simulink library "AFS_MasterFeature"  (R2020b)
settings: Solver=FixedStepDiscrete  StartTime=0.0  StopTime=10.0  FixedStep=SampleTime  RelTol=1e-3
undefined symbols (not defined in the file): C_AFS_Thr_Speed_HB_HS_OFF, C_AFS_Thr_Speed_HB_HS_ON, C_F_SpeedCountry2Town, C_F_SpeedPed2Town, C_F_SpeedTown2Country, C_F_SpeedTown2Ped, C_F_Time2WaitAFS, C_ParkingSpeedThrAct, C_SpeedCountry2MW, C_SpeedMW2Country, C_TeAfsMaster, C_TempoPark, N_E_AdverseWeather, N_E_Country, N_E_Foggy, N_E_HBHighSpeed, N_E_HBLowSpeed, N_E_Motorway, N_E_NoFunction, N_E_Pedestrian, N_E_TouristMode, N_E_Town, N_LIGHT_NIGHT, N_ManeuverMode
settings Model: Creator=hhamlaou  LastModifiedBy=smettupa
settings DataIOCC: ReturnWorkspaceOutputs=off
settings DebuggingCC: ArithmeticOperatorsInVariantConditions=warning
settings SFSimCC: SimUseLocalCustomCode=off  CustomCodeUndefinedFunction=UseInterfaceOnly
settings RTWCC: RTWUseLocalCustomCode=off

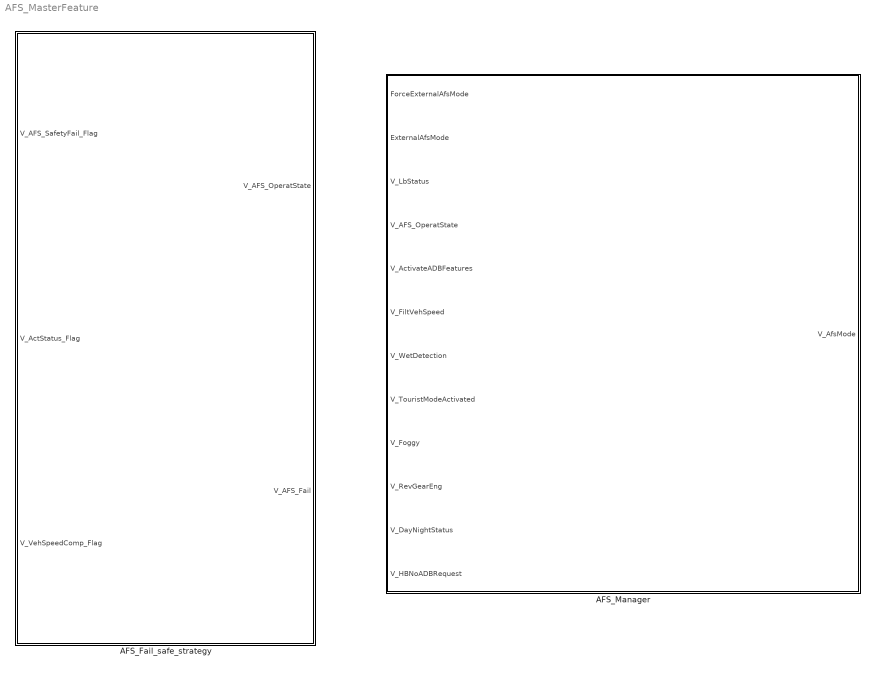
== system AFS_MasterFeature ==
  AFS_Fail_safe_strategy : Stateflow chart  TreatAsAtomicUnit=on
  AFS_Manager : Subsystem  Description=AFS_Subsystem

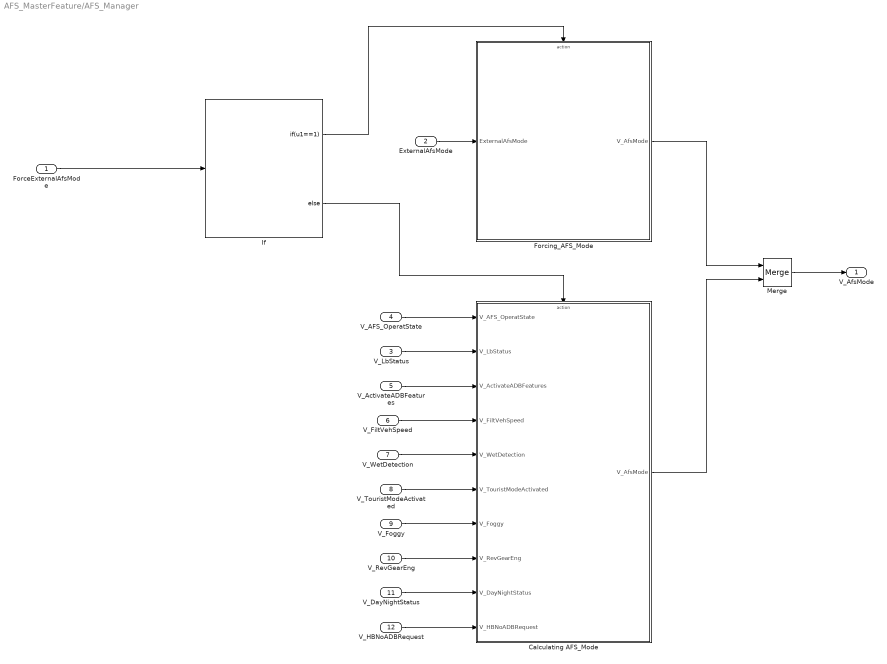
== system AFS_MasterFeature/AFS_Manager ==
  ForceExternalAfsMode : Inport
  ExternalAfsMode : Inport  Port=2
  V_LbStatus : Inport  Port=3
  V_AFS_OperatState : Inport  Port=4
  V_ActivateADBFeatures : Inport  Port=5
  V_FiltVehSpeed : Inport  Port=6
  V_WetDetection : Inport  Port=7
  V_TouristModeActivated : Inport  Port=8
  V_Foggy : Inport  Port=9
  V_RevGearEng : Inport  Port=10
  V_DayNightStatus : Inport  Port=11
  V_HBNoADBRequest : Inport  Port=12
  "Calculating AFS_Mode " : Subsystem  TreatAsAtomicUnit=on
  Forcing_AFS_Mode : Subsystem  TreatAsAtomicUnit=on
  If : If  IfExpression=u1==1
  Merge : Merge
  V_AfsMode : Outport
  wires:
  ForceExternalAfsMode/1 -> If/1
  Forcing_AFS_Mode/1(V_AfsMode) -> Merge/1
  "Calculating AFS_Mode "/1(V_AfsMode) -> Merge/2
  Merge/1 -> V_AfsMode/1
  ExternalAfsMode/1 -> Forcing_AFS_Mode/1(ExternalAfsMode)
  V_LbStatus/1 -> "Calculating AFS_Mode "/2(V_LbStatus)
  V_AFS_OperatState/1 -> "Calculating AFS_Mode "/1(V_AFS_OperatState)
  V_ActivateADBFeatures/1 -> "Calculating AFS_Mode "/3(V_ActivateADBFeatures)
  V_FiltVehSpeed/1 -> "Calculating AFS_Mode "/4(V_FiltVehSpeed)
  V_WetDetection/1 -> "Calculating AFS_Mode "/5(V_WetDetection)
  V_TouristModeActivated/1 -> "Calculating AFS_Mode "/6(V_TouristModeActivated)
  V_Foggy/1 -> "Calculating AFS_Mode "/7(V_Foggy)
  V_RevGearEng/1 -> "Calculating AFS_Mode "/8(V_RevGearEng)
  V_DayNightStatus/1 -> "Calculating AFS_Mode "/9(V_DayNightStatus)
  If/1 -> Forcing_AFS_Mode/Action
  V_HBNoADBRequest/1 -> "Calculating AFS_Mode "/10(V_HBNoADBRequest)
  If/2 -> "Calculating AFS_Mode "/Action

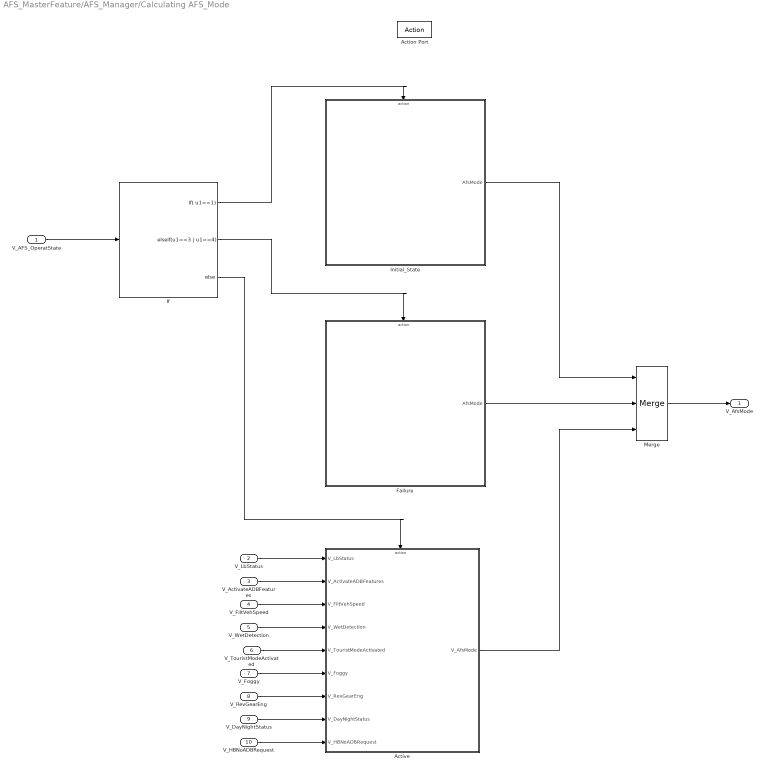
== system AFS_MasterFeature/AFS_Manager/Calculating AFS_Mode  ==
  V_AFS_OperatState : Inport
  V_LbStatus : Inport  Port=2
  V_ActivateADBFeatures : Inport  Port=3
  V_FiltVehSpeed : Inport  Port=4
  V_WetDetection : Inport  Port=5
  V_TouristModeActivated : Inport  Port=6
  V_Foggy : Inport  Port=7
  V_RevGearEng : Inport  Port=8
  V_DayNightStatus : Inport  Port=9
  V_HBNoADBRequest : Inport  Port=10
  Action Port : ActionPort
  Active : Subsystem  TreatAsAtomicUnit=on
  Failure : Subsystem  TreatAsAtomicUnit=on
  If : If  IfExpression=u1==1  ElseIfExpressions=u1==3 | u1==4
  Initial_State : Subsystem  TreatAsAtomicUnit=on
  Merge : Merge  Inputs=3
  V_AfsMode : Outport
  wires:
  V_AFS_OperatState/1 -> If/1
  If/2 -> Failure/Action
  If/3 -> Active/Action
  Failure/1(AfsMode) -> Merge/2
  Initial_State/1(AfsMode) -> Merge/1
  Active/1(V_AfsMode) -> Merge/3
  Merge/1 -> V_AfsMode/1
  V_ActivateADBFeatures/1 -> Active/2(V_ActivateADBFeatures)
  V_LbStatus/1 -> Active/1(V_LbStatus)
  V_FiltVehSpeed/1 -> Active/3(V_FiltVehSpeed)
  V_WetDetection/1 -> Active/4(V_WetDetection)
  V_TouristModeActivated/1 -> Active/5(V_TouristModeActivated)
  V_Foggy/1 -> Active/6(V_Foggy)
  V_RevGearEng/1 -> Active/7(V_RevGearEng)
  V_DayNightStatus/1 -> Active/8(V_DayNightStatus)
  V_HBNoADBRequest/1 -> Active/9(V_HBNoADBRequest)
  If/1 -> Initial_State/Action

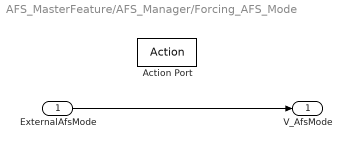
== system AFS_MasterFeature/AFS_Manager/Forcing_AFS_Mode ==
  ExternalAfsMode : Inport
  Action Port : ActionPort
  V_AfsMode : Outport
  wires:
  ExternalAfsMode/1 -> V_AfsMode/1

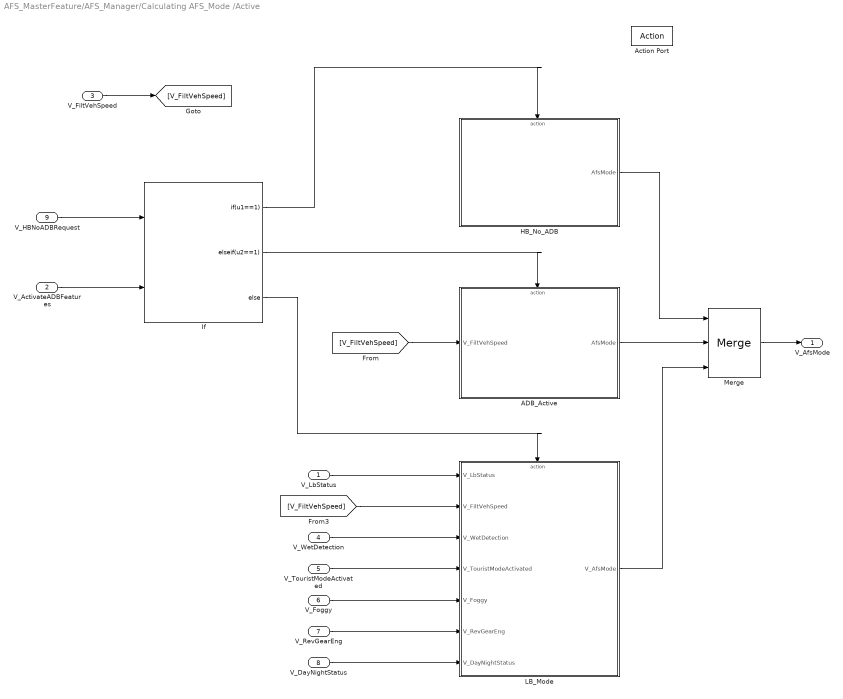
== system AFS_MasterFeature/AFS_Manager/Calculating AFS_Mode /Active ==
  V_LbStatus : Inport
  V_ActivateADBFeatures : Inport  Port=2
  V_FiltVehSpeed : Inport  Port=3
  V_WetDetection : Inport  Port=4
  V_TouristModeActivated : Inport  Port=5
  V_Foggy : Inport  Port=6
  V_RevGearEng : Inport  Port=7
  V_DayNightStatus : Inport  Port=8
  V_HBNoADBRequest : Inport  Port=9
  Action Port : ActionPort
  ADB_Active : Subsystem  TreatAsAtomicUnit=on
  HB_No_ADB : Subsystem  TreatAsAtomicUnit=on
  If : If  NumInputs=2  IfExpression=u1==1  ElseIfExpressions=u2==1
  LB_Mode : Subsystem  TreatAsAtomicUnit=on
  Merge : Merge  Inputs=3
  V_AfsMode : Outport
  wires:
  V_FiltVehSpeed/1 -> [V_FiltVehSpeed]
  V_HBNoADBRequest/1 -> If/1
  If/1 -> HB_No_ADB/Action
  V_ActivateADBFeatures/1 -> If/2
  If/2 -> ADB_Active/Action
  If/3 -> LB_Mode/Action
  ADB_Active/1(AfsMode) -> Merge/2
  HB_No_ADB/1(AfsMode) -> Merge/1
  LB_Mode/1(V_AfsMode) -> Merge/3
  [V_FiltVehSpeed] -> ADB_Active/1(V_FiltVehSpeed)
  Merge/1 -> V_AfsMode/1
  V_LbStatus/1 -> LB_Mode/1(V_LbStatus)
  [V_FiltVehSpeed] -> LB_Mode/2(V_FiltVehSpeed)
  V_WetDetection/1 -> LB_Mode/3(V_WetDetection)
  V_TouristModeActivated/1 -> LB_Mode/4(V_TouristModeActivated)
  V_Foggy/1 -> LB_Mode/5(V_Foggy)
  V_RevGearEng/1 -> LB_Mode/6(V_RevGearEng)
  V_DayNightStatus/1 -> LB_Mode/7(V_DayNightStatus)

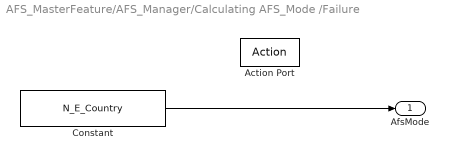
== system AFS_MasterFeature/AFS_Manager/Calculating AFS_Mode /Failure ==
  Action Port : ActionPort
  Constant : Constant  Value=N_E_Country
  AfsMode : Outport
  wires:
  Constant/1 -> AfsMode/1

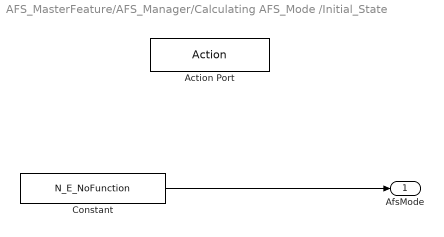
== system AFS_MasterFeature/AFS_Manager/Calculating AFS_Mode /Initial_State ==
  Action Port : ActionPort
  Constant : Constant  Value=N_E_NoFunction
  AfsMode : Outport
  wires:
  Constant/1 -> AfsMode/1

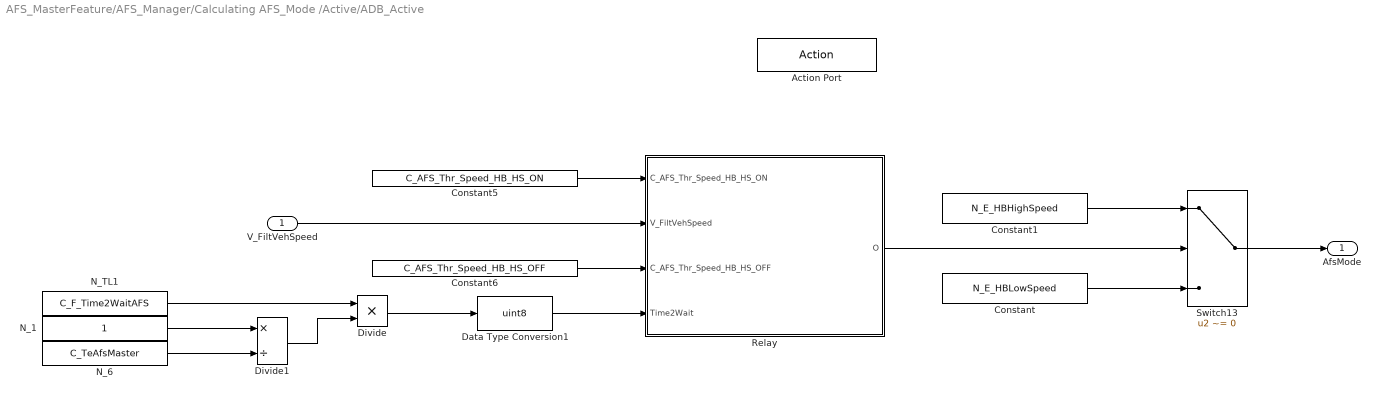
== system AFS_MasterFeature/AFS_Manager/Calculating AFS_Mode /Active/ADB_Active ==
  V_FiltVehSpeed : Inport
  Action Port : ActionPort
  Constant : Constant  Value=N_E_HBLowSpeed
  Constant1 : Constant  Value=N_E_HBHighSpeed
  Constant5 : Constant  Value=C_AFS_Thr_Speed_HB_HS_ON
  Constant6 : Constant  Value=C_AFS_Thr_Speed_HB_HS_OFF
  Data Type Conversion1 : DataTypeConversion  OutDataTypeStr=uint8
  Divide : Product  Inputs=**
  Divide1 : Product  Inputs=*/  OutDataTypeStr=uint8
  N_1 : Constant  OutDataTypeStr=uint8
  N_6 : Constant  Value=C_TeAfsMaster
  N_TL1 : Constant  Value=C_F_Time2WaitAFS
  Relay : Stateflow chart  TreatAsAtomicUnit=on
  Switch13 : Switch  Criteria=u2 ~= 0
  AfsMode : Outport
  wires:
  V_FiltVehSpeed/1 -> Relay/2(V_FiltVehSpeed)
  Data Type Conversion1/1 -> Relay/4(Time2Wait)
  Constant5/1 -> Relay/1(C_AFS_Thr_Speed_HB_HS_ON)
  Constant6/1 -> Relay/3(C_AFS_Thr_Speed_HB_HS_OFF)
  Relay/1(O) -> Switch13/2
  Constant1/1 -> Switch13/1
  Constant/1 -> Switch13/3
  Switch13/1 -> AfsMode/1
  N_1/1 -> Divide1/1
  Divide/1 -> Data Type Conversion1/1
  N_TL1/1 -> Divide/1
  Divide1/1 -> Divide/2
  N_6/1 -> Divide1/2

== system AFS_MasterFeature/AFS_Manager/Calculating AFS_Mode /Active/HB_No_ADB ==
  Action Port : ActionPort
  Constant : Constant  Value=N_E_HBLowSpeed
  AfsMode : Outport
  wires:
  Constant/1 -> AfsMode/1

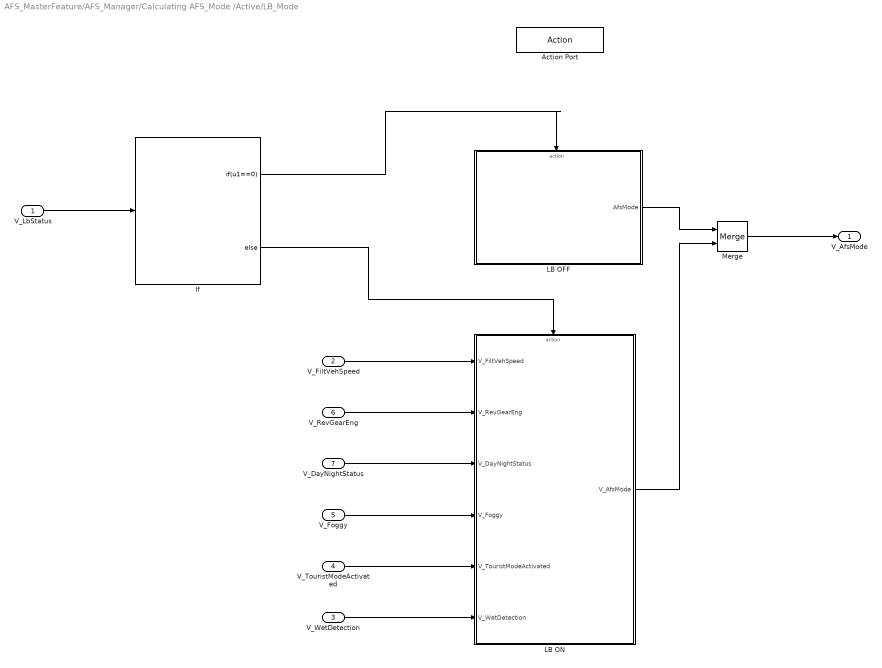
== system AFS_MasterFeature/AFS_Manager/Calculating AFS_Mode /Active/LB_Mode ==
  V_LbStatus : Inport
  V_FiltVehSpeed : Inport  Port=2
  V_WetDetection : Inport  Port=3
  V_TouristModeActivated : Inport  Port=4
  V_Foggy : Inport  Port=5
  V_RevGearEng : Inport  Port=6
  V_DayNightStatus : Inport  Port=7
  Action Port : ActionPort
  If : If  IfExpression=u1==0
  LB OFF : Subsystem  TreatAsAtomicUnit=on
  LB ON : Subsystem  TreatAsAtomicUnit=on
  Merge : Merge
  V_AfsMode : Outport
  wires:
  If/1 -> LB OFF/Action
  If/2 -> LB ON/Action
  LB OFF/1(AfsMode) -> Merge/1
  LB ON/1(V_AfsMode) -> Merge/2
  Merge/1 -> V_AfsMode/1
  V_FiltVehSpeed/1 -> LB ON/1(V_FiltVehSpeed)
  V_LbStatus/1 -> If/1
  V_RevGearEng/1 -> LB ON/2(V_RevGearEng)
  V_DayNightStatus/1 -> LB ON/3(V_DayNightStatus)
  V_Foggy/1 -> LB ON/4(V_Foggy)
  V_TouristModeActivated/1 -> LB ON/5(V_TouristModeActivated)
  V_WetDetection/1 -> LB ON/6(V_WetDetection)

== system AFS_MasterFeature/AFS_Manager/Calculating AFS_Mode /Active/LB_Mode/LB OFF ==
  Action Port : ActionPort
  Constant : Constant  Value=N_E_NoFunction
  AfsMode : Outport
  wires:
  Constant/1 -> AfsMode/1

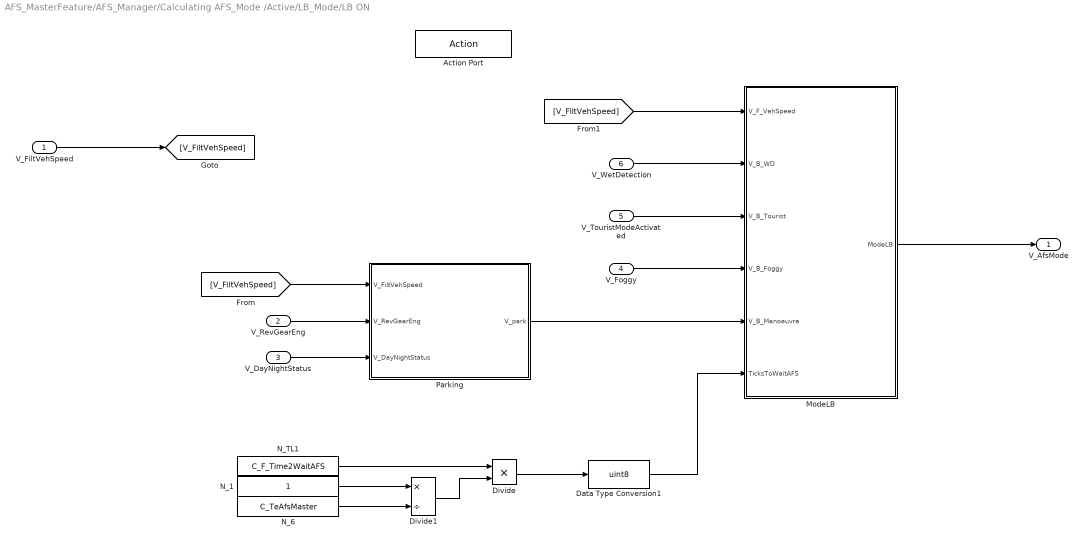
== system AFS_MasterFeature/AFS_Manager/Calculating AFS_Mode /Active/LB_Mode/LB ON ==
  V_FiltVehSpeed : Inport
  V_RevGearEng : Inport  Port=2
  V_DayNightStatus : Inport  Port=3
  V_Foggy : Inport  Port=4
  V_TouristModeActivated : Inport  Port=5
  V_WetDetection : Inport  Port=6
  Action Port : ActionPort
  Data Type Conversion1 : DataTypeConversion  OutDataTypeStr=uint8
  Divide : Product  Inputs=**
  Divide1 : Product  Inputs=*/  OutDataTypeStr=uint8
  ModeLB : Subsystem  Description=ModeLB
  N_1 : Constant  OutDataTypeStr=uint8
  N_6 : Constant  Value=C_TeAfsMaster
  N_TL1 : Constant  Value=C_F_Time2WaitAFS
  Parking : Subsystem  TreatAsAtomicUnit=on
  V_AfsMode : Outport
  wires:
  Parking/1(V_park) -> ModeLB/5(V_B_Manoeuvre)
  N_TL1/1 -> Divide/1
  Data Type Conversion1/1 -> ModeLB/6(TicksToWaitAFS)
  N_6/1 -> Divide1/2
  Divide/1 -> Data Type Conversion1/1
  Divide1/1 -> Divide/2
  N_1/1 -> Divide1/1
  ModeLB/1(ModeLB) -> V_AfsMode/1
  V_RevGearEng/1 -> Parking/2(V_RevGearEng)
  V_DayNightStatus/1 -> Parking/3(V_DayNightStatus)
  V_Foggy/1 -> ModeLB/4(V_B_Foggy)
  V_TouristModeActivated/1 -> ModeLB/3(V_B_Tourist)
  V_WetDetection/1 -> ModeLB/2(V_B_WD)
  V_FiltVehSpeed/1 -> [V_FiltVehSpeed]
  [V_FiltVehSpeed] -> Parking/1(V_FiltVehSpeed)
  [V_FiltVehSpeed] -> ModeLB/1(V_F_VehSpeed)

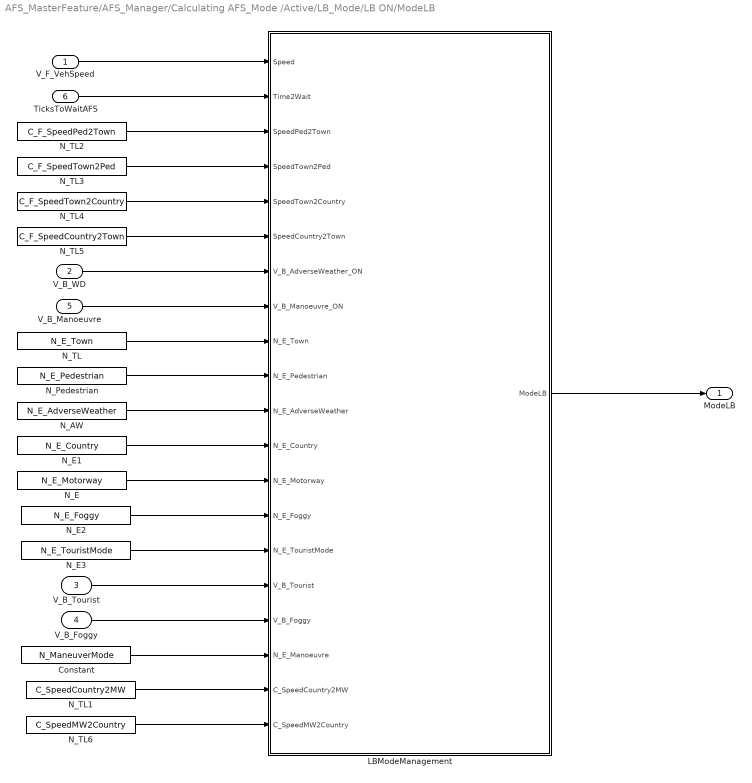
== system AFS_MasterFeature/AFS_Manager/Calculating AFS_Mode /Active/LB_Mode/LB ON/ModeLB ==
  V_F_VehSpeed : Inport
  V_B_WD : Inport  Port=2
  V_B_Tourist : Inport  Port=3
  V_B_Foggy : Inport  Port=4
  V_B_Manoeuvre : Inport  Port=5
  TicksToWaitAFS : Inport  Port=6
      settings: AttributesFormatString=%<OutDataTypeStr>
  Constant : Constant  Value=N_ManeuverMode
  LBModeManagement : Stateflow chart
  N_AW : Constant  Value=N_E_AdverseWeather
  N_E : Constant  Value=N_E_Motorway
  N_E1 : Constant  Value=N_E_Country
  N_E2 : Constant  Value=N_E_Foggy
  N_E3 : Constant  Value=N_E_TouristMode
  N_Pedestrian : Constant  Value=N_E_Pedestrian
  N_TL : Constant  Value=N_E_Town
  N_TL1 : Constant  Value=C_SpeedCountry2MW
  N_TL2 : Constant  Value=C_F_SpeedPed2Town
  N_TL3 : Constant  Value=C_F_SpeedTown2Ped
  N_TL4 : Constant  Value=C_F_SpeedTown2Country
  N_TL5 : Constant  Value=C_F_SpeedCountry2Town
  N_TL6 : Constant  Value=C_SpeedMW2Country
  ModeLB : Outport  VectorParamsAs1DForOutWhenUnconnected=off
  wires:
  N_TL4/1 -> LBModeManagement/5(SpeedTown2Country)
  N_TL3/1 -> LBModeManagement/4(SpeedTown2Ped)
  V_F_VehSpeed/1 -> LBModeManagement/1(Speed)
  LBModeManagement/1(ModeLB) -> ModeLB/1
  N_TL2/1 -> LBModeManagement/3(SpeedPed2Town)
  N_TL5/1 -> LBModeManagement/6(SpeedCountry2Town)
  V_B_WD/1 -> LBModeManagement/7(V_B_AdverseWeather_ON)
  N_AW/1 -> LBModeManagement/11(N_E_AdverseWeather)
  N_Pedestrian/1 -> LBModeManagement/10(N_E_Pedestrian)
  N_E/1 -> LBModeManagement/13(N_E_Motorway)
  N_E1/1 -> LBModeManagement/12(N_E_Country)
  N_TL/1 -> LBModeManagement/9(N_E_Town)
  N_E2/1 -> LBModeManagement/14(N_E_Foggy)
  N_E3/1 -> LBModeManagement/15(N_E_TouristMode)
  V_B_Tourist/1 -> LBModeManagement/16(V_B_Tourist)
  V_B_Foggy/1 -> LBModeManagement/17(V_B_Foggy)
  TicksToWaitAFS/1 -> LBModeManagement/2(Time2Wait)
  V_B_Manoeuvre/1 -> LBModeManagement/8(V_B_Manoeuvre_ON)
  Constant/1 -> LBModeManagement/18(N_E_Manoeuvre)
  N_TL1/1 -> LBModeManagement/19(C_SpeedCountry2MW)
  N_TL6/1 -> LBModeManagement/20(C_SpeedMW2Country)

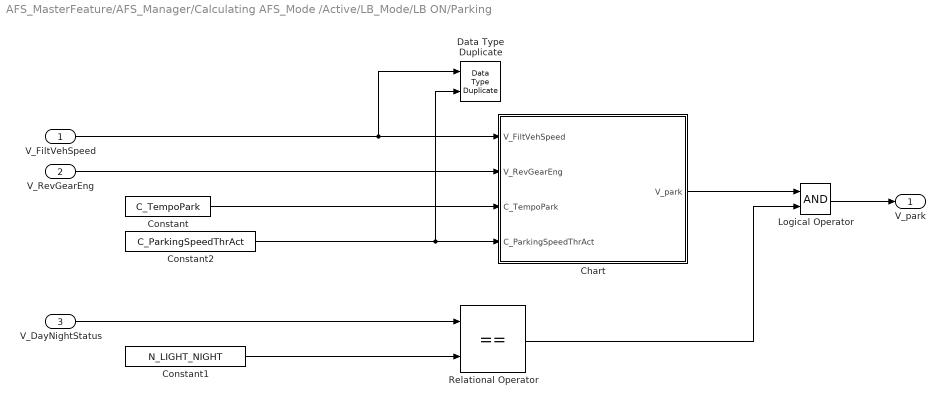
== system AFS_MasterFeature/AFS_Manager/Calculating AFS_Mode /Active/LB_Mode/LB ON/Parking ==
  V_FiltVehSpeed : Inport
  V_RevGearEng : Inport  Port=2
  V_DayNightStatus : Inport  Port=3
  Chart : Stateflow chart  TreatAsAtomicUnit=on
  Constant : Constant  Value=C_TempoPark
  Constant1 : Constant  Value=N_LIGHT_NIGHT
  Constant2 : Constant  Value=C_ParkingSpeedThrAct
  Data Type Duplicate : DataTypeDuplicate
  Logical Operator : Logic  AllPortsSameDT=off  OutDataTypeStr=boolean
  Relational Operator : RelationalOperator  Operator===  OutDataTypeStr=boolean  RndMeth=Simplest
  V_park : Outport  VectorParamsAs1DForOutWhenUnconnected=off
  wires:
  Chart/1(V_park) -> Logical Operator/1
  Logical Operator/1 -> V_park/1
  Constant1/1 -> Relational Operator/2
  Relational Operator/1 -> Logical Operator/2
  Constant/1 -> Chart/3(C_TempoPark)
  Constant2/1 -> Chart/4(C_ParkingSpeedThrAct), Data Type Duplicate/2
  V_FiltVehSpeed/1 -> Data Type Duplicate/1, Chart/1(V_FiltVehSpeed)
  V_DayNightStatus/1 -> Relational Operator/1
  V_RevGearEng/1 -> Chart/2(V_RevGearEng)

== stateflow chart AFS_MasterFeature/AFS_Fail_safe_strategy ==
  state Init_system
    entry:
    V_AFS_OperatState = 1;
    V_AFS_Fail = 0;
  state FSM_AFS_safety
    entry:
    V_AFS_OperatState = 4;
    V_AFS_Fail = 1;
  state AFS_function_active
    entry:
    V_AFS_OperatState = 2;
    V_AFS_Fail = 0;
  state AFS_Freeze
    entry:
    V_AFS_OperatState =3;
  (default) -> Init_system
  Init_system -> FSM_AFS_safety [order 1] : [V_AFS_SafetyFail_Flag==1]
  Init_system -> AFS_function_active [order 3] : [(V_VehSpeedComp_Flag==1)]
  Init_system -> AFS_Freeze [order 2] : [(V_ActStatus_Flag==0)]
  FSM_AFS_safety -> AFS_function_active : [(V_ActStatus_Flag== 1)...
      | &&(V_VehSpeedComp_Flag== 1)...
      | &&(V_AFS_SafetyFail_Flag == 0)]
  AFS_function_active -> FSM_AFS_safety [order 1] : [V_AFS_SafetyFail_Flag ==1]
  AFS_Freeze -> FSM_AFS_safety [order 1] : [V_AFS_SafetyFail_Flag ==1]
  AFS_function_active -> AFS_Freeze [order 2] : [(V_ActStatus_Flag== 0)]
  AFS_Freeze -> AFS_function_active [order 2] : [(V_ActStatus_Flag== 1)...
      | &&(V_VehSpeedComp_Flag== 1)]
  data: V_AFS_OperatState output uint8; V_AFS_Fail output boolean; V_AFS_SafetyFail_Flag input boolean; V_ActStatus_Flag input boolean; V_VehSpeedComp_Flag input boolean
  data V_AFS_OperatState settings: description=$TL$ type=UInt8; $TL$

== stateflow chart AFS_MasterFeature/AFS_Manager/Calculating AFS_Mode /Active/LB_Mode/LB ON/ModeLB/LBModeManagement ==
  state LBActivated
    state Pedestrian
      en:
      ModeLB=N_E_Pedestrian;
    state Ped2Town
    state Town
      en:
      ModeLB=N_E_Town;
    state Town2Ped
    state Country2Town
    state Country
      en:
      ModeLB=N_E_Country;
    state Town2Country
    state Country2MW
    state MotorwayLB
      en:
      ModeLB=N_E_Motorway;
    state MW2Country
    (default) -> (junction 67)
    (junction 67) -> (junction 68) [order 1] : [Speed<SpeedTown2Country]
    (junction 68) -> Pedestrian [order 1] : [Speed<SpeedPed2Town]
    (junction 68) -> Town [order 2]
    (junction 67) -> Country [order 2]
    Ped2Town -> Pedestrian [order 2] : [Speed<SpeedPed2Town]
    Pedestrian -> Ped2Town : [Speed>=SpeedPed2Town]
    Ped2Town -> Town [order 1] : [after(Time2Wait,tick)]
    Town2Ped -> Pedestrian [order 2] : [after(Time2Wait,tick)]
    Town2Ped -> Town [order 1] : [Speed>SpeedTown2Ped]
    Town -> Town2Ped [order 1] : [Speed<=SpeedTown2Ped]
    Country2Town -> Town [order 1] : [after(Time2Wait,tick)]
    Country -> Country2Town [order 1] : [Speed<=SpeedCountry2Town]
    Country2Town -> Country [order 2] : [Speed>SpeedCountry2Town]
    Town -> Town2Country [order 2] : [Speed>=SpeedTown2Country]
    Town2Country -> Town [order 1] : [Speed<SpeedTown2Country]
    Country -> Country2MW [order 2] : [Speed>C_SpeedCountry2MW]
    Town2Country -> Country [order 2] : [after(Time2Wait,tick)]
    Country2MW -> Country [order 2] : [Speed<=C_SpeedMW2Country]
    Country2MW -> MotorwayLB [order 1] : [after(Time2Wait,tick)]
    MW2Country -> Country [order 1] : [after(Time2Wait,tick)]
    MotorwayLB -> MW2Country : [Speed<=C_SpeedMW2Country]
    MW2Country -> MotorwayLB [order 2] : [Speed>C_SpeedCountry2MW]
  state Maneuvre
    en:
    ModeLB=N_E_Manoeuvre;
  state AdverseWeather
    en:
    ModeLB=N_E_AdverseWeather;
  state Tourist
    en:
    ModeLB=N_E_TouristMode;
  state Fog
    en:
    ModeLB=N_E_Foggy;
  (default) -> LBActivated
  LBActivated -> Maneuvre [order 1] : [V_B_Manoeuvre_ON]
  Maneuvre -> LBActivated : [!V_B_Manoeuvre_ON]
  LBActivated -> AdverseWeather [order 4] : [V_B_AdverseWeather_ON]
  AdverseWeather -> LBActivated : [!V_B_AdverseWeather_ON]
  LBActivated -> Tourist [order 2] : [V_B_Tourist]
  Tourist -> LBActivated : [!V_B_Tourist]
  LBActivated -> Fog [order 3] : [V_B_Foggy]
  Fog -> LBActivated : [!V_B_Foggy]
  data: Speed input; ModeLB output uint8; Time2Wait input; SpeedPed2Town input; SpeedTown2Ped input; SpeedTown2Country input; SpeedCountry2Town input; V_B_AdverseWeather_ON input; V_B_Manoeuvre_ON input; N_E_Town input; N_E_Pedestrian input; N_E_AdverseWeather input; N_E_Country input; N_E_Motorway input; N_E_Foggy input; N_E_TouristMode input; V_B_Tourist input; V_B_Foggy input; N_E_Manoeuvre input; C_SpeedCountry2MW input; C_SpeedMW2Country input

== stateflow chart AFS_MasterFeature/AFS_Manager/Calculating AFS_Mode /Active/ADB_Active/Relay ==
  state OFF
    en:
    O=0;
  state Waiting1
  state Waiting
  state ON
    en:
    O=1;
  (default) -> OFF
  Waiting1 -> OFF [order 2] : [after(Time2Wait,tick)]
  Waiting -> OFF [order 2] : [V_FiltVehSpeed<=C_AFS_Thr_Speed_HB_HS_ON]
  OFF -> Waiting : [V_FiltVehSpeed > C_AFS_Thr_Speed_HB_HS_ON]
  Waiting1 -> ON [order 1] : [V_FiltVehSpeed > C_AFS_Thr_Speed_HB_HS_OFF]
  ON -> Waiting1 : [V_FiltVehSpeed <= C_AFS_Thr_Speed_HB_HS_OFF]
  Waiting -> ON [order 1] : [after(Time2Wait,tick)]
  data: C_AFS_Thr_Speed_HB_HS_ON input; V_FiltVehSpeed input; C_AFS_Thr_Speed_HB_HS_OFF input; O output boolean; Time2Wait input

== stateflow chart AFS_MasterFeature/AFS_Manager/Calculating AFS_Mode /Active/LB_Mode/LB ON/Parking/Chart ==
  state park_situation
    state d
      entry:
      V_park=0;
    state a
    state b
      entry:
      V_park=1;
    state c
      entry:
      V_park=0;
    (default) -> d
    d -> a : [(V_RevGearEng == 1) && (V_FiltVehSpeed < C_ParkingSpeedThrAct)]
    a -> (junction 13) [order 1] : [(V_FiltVehSpeed > C_ParkingSpeedThrAct)]
    a -> b [order 2] : [(V_RevGearEng == 0) && (V_FiltVehSpeed < C_ParkingSpeedThrAct)]
    (junction 13) -> d
    b -> c : [after(C_TempoPark,tick) || (V_FiltVehSpeed > C_ParkingSpeedThrAct)]
    c -> (junction 13)
  data: V_park output boolean; V_FiltVehSpeed input; V_RevGearEng input; C_TempoPark input; C_ParkingSpeedThrAct input
